simulink model "sfcndemo_sfun_zc_sat"  (Simulink 6.0)
settings: Solver=FixedStepDiscrete  SolverMode=SingleTasking  StartTime=0.0  StopTime=10.0  RelTol=1e-3
settings Model: Creator=The MathWorks Inc.  LastModifiedBy=batserve  ExtModeTrigMode=oneshot  ExtModeArmWhenConnect=off  ExtModeAutoUpdateStatusClock=off
settings DataIOCC: LimitDataPoints=off
settings OptimizationCC: BooleanDataType=off
settings DebuggingCC: CheckExecutionContextPreStartOutputMsg=on  CheckExecutionContextRuntimeOutputMsg=on  SolverPrmCheckMsg=none  InheritedTsInSrcMsg=none
settings HardwareCC: TargetUnknown=on

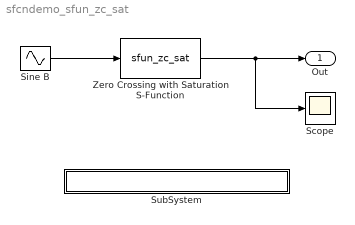
== system sfcndemo_sfun_zc_sat ==
  Scope : Scope
      settings: TimeRange=10  YMin=-0.5  YMax=1  SampleInput=on  SampleTime=-1
  Sine B : Sin
  SubSystem : Subsystem  PropExecContextAcrossSSBoundary=on
      settings: OpenFcn=edit(fullfile(matlabroot,'simulink','src','sfun_zc_sat.c'))
      mask Display: disp('matlabroot\simulink\src\sfun_zc_sat.c');
  Zero Crossing with Saturation S-Function : S-Function  FunctionName=sfun_zc_sat  Parameters=ub, lb  mask(S-function: sfun_zc_sat){ub=[0.5 0.75], lb=[0,-.5]}
      mask prompts: ub "Upper Limit"; lb "Lower Limit"
      mask help: This is a S-function block which has nonsampled zero crossings to implement a saturation function.
  Out : Outport  InitialOutput=0
  wires:
  Sine B/1 -> Zero Crossing with Saturation S-Function/1
  Zero Crossing with Saturation S-Function/1 -> Out/1, Scope/1

== system sfcndemo_sfun_zc_sat/SubSystem ==
